simulink model "LaborDaySim"  (R2012b)
settings: Solver=ode45  StartTime=0.0  StopTime=20.0  RelTol=1e-3
libraries: simulink x3
settings Model: Creator=Kushal  LastModifiedBy=Kushal

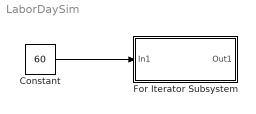
== system LaborDaySim ==
  Constant : Constant  Value=60
  For Iterator Subsystem : Subsystem  TreatAsAtomicUnit=on
  wires:
  Constant/1 -> For Iterator Subsystem/1(In1)

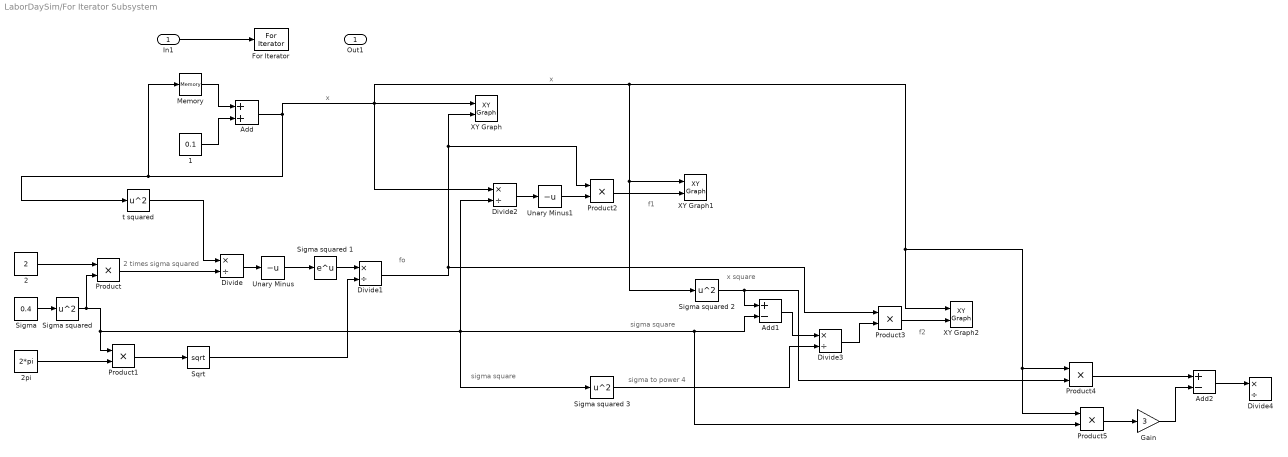
== system LaborDaySim/For Iterator Subsystem ==
  note: f2
  note: sigma to power 4
  note: sigma square
  note: sigma square
  note: x square
  note: x
  note: x
  note: f1
  note: fo
  note: 2 times sigma squared
  In1 : Inport
  1 : Constant  Value=0.1
  2 : Constant  Value=2
  "2pi " : Constant  Value=2*pi
  Add : Sum
  Add1 : Sum  Inputs=+-
  Add2 : Sum  Inputs=+-
  Divide{,1..4} (5 alike) : Product  Inputs=*/
  For Iterator : ForIterator  ResetStates=reset  IterationSource=external
  Gain : Gain  Gain=3
  Memory : Memory  X0=-3.1  InheritSampleTime=on
  Product{,1..5} (6 alike) : Product  RndMeth=Zero
  "Sigma " : Constant  Value=0.4
  "Sigma squared " : Math  Operator=square  SaturateOnIntegerOverflow=on
  Sigma squared 1 : Math  SaturateOnIntegerOverflow=on
  Sigma squared 2 : Math  Operator=square  SaturateOnIntegerOverflow=on
  Sigma squared 3 : Math  Operator=square  SaturateOnIntegerOverflow=on
  Sqrt : Sqrt  SaturateOnIntegerOverflow=on
  Unary Minus : UnaryMinus
  Unary Minus1 : UnaryMinus
  XY Graph : simulink/Sinks/XY Graph  xmin=-3  xmax=3  ymin=0  ymax=1  st=-1
  XY Graph1 : simulink/Sinks/XY Graph  xmin=-3  xmax=3  ymin=-1.6  ymax=1.6  st=-1
  XY Graph2 : simulink/Sinks/XY Graph  xmin=-3  xmax=3  ymin=-6.5  ymax=3  st=-1
  "t squared " : Math  Operator=square  SaturateOnIntegerOverflow=on
  Out1 : Outport
  wires:
  "Sigma "/1 -> "Sigma squared "/1
  "t squared "/1 -> Divide/1
  Product/1 -> Divide/2
  Sigma squared 1/1 -> Divide1/1
  2/1 -> Product/1
  "Sigma squared "/1 -> Product5/2, Add1/2, Divide2/2, Sigma squared 3/1, Product1/1, Product/2
  "2pi "/1 -> Product1/2
  Product1/1 -> Sqrt/1
  Sqrt/1 -> Divide1/2
  Unary Minus/1 -> Sigma squared 1/1
  Divide/1 -> Unary Minus/1
  In1/1 -> For Iterator/1
  Memory/1 -> Add/1
  1/1 -> Add/2
  Divide1/1 -> Product3/1, XY Graph/2, Product2/1
  Add/1 -> "t squared "/1, Memory/1, Sigma squared 2/1, XY Graph1/1, XY Graph2/1, Product5/1, Product4/1, Divide2/1, XY Graph/1
  Divide2/1 -> Unary Minus1/1
  Unary Minus1/1 -> Product2/2
  Product2/1 -> XY Graph1/2
  Sigma squared 2/1 -> Product4/2, Add1/1
  Add1/1 -> Divide3/1
  Sigma squared 3/1 -> Divide3/2
  Divide3/1 -> Product3/2
  Product3/1 -> XY Graph2/2
  Product4/1 -> Add2/1
  Product5/1 -> Gain/1
  Gain/1 -> Add2/2
  Add2/1 -> Divide4/1
